simulink model "stereo_ibvs_ros2_stage1"  (R2025b)
settings: Solver=FixedStepDiscrete  StartTime=0  StopTime=inf  FixedStep=cfg.Ts  RelTol=1e-3
PostLoadFcn:
  | wrapperFile__=get_param(bdroot,'FileName');ros2Dir__=fileparts(wrapperFile__);simulinkDir__=fileparts(ros2Dir__);coreDir__=fullfile(simulinkDir__,'core');configDir__=fullfile(simulinkDir__,'config');addpath(coreDir__);addpath(configDir__);run(fullfile(configDir__,'stereo_ibvs_config.m'));clear wrapperFile__ ros2Dir__ simulinkDir__ coreDir__ configDir__;
InitFcn:
  | wrapperFile__=get_param(bdroot,'FileName');ros2Dir__=fileparts(wrapperFile__);simulinkDir__=fileparts(ros2Dir__);coreDir__=fullfile(simulinkDir__,'core');configDir__=fullfile(simulinkDir__,'config');addpath(coreDir__);addpath(configDir__);run(fullfile(configDir__,'stereo_ibvs_config.m'));clear wrapperFile__ ros2Dir__ simulinkDir__ coreDir__ configDir__;
undefined symbols (not defined in the file): cfg, data, data_SL_Info
libraries: ros2lib x10, simulink x3
settings Model: Creator=hlc  LastModifiedBy=hlc
settings DataIOCC: SignalLogging=off  SaveTime=off

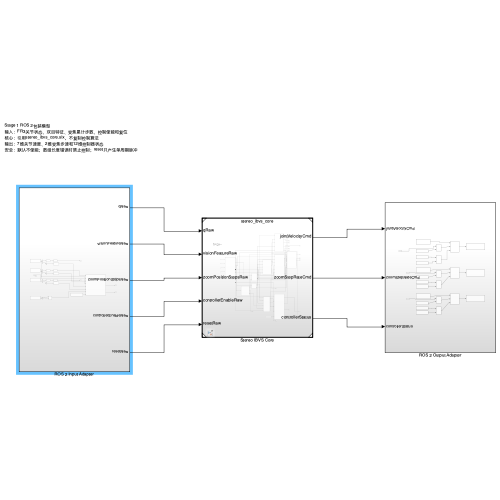
[thumbnail: Simulink's stored preview of the top-level diagram]
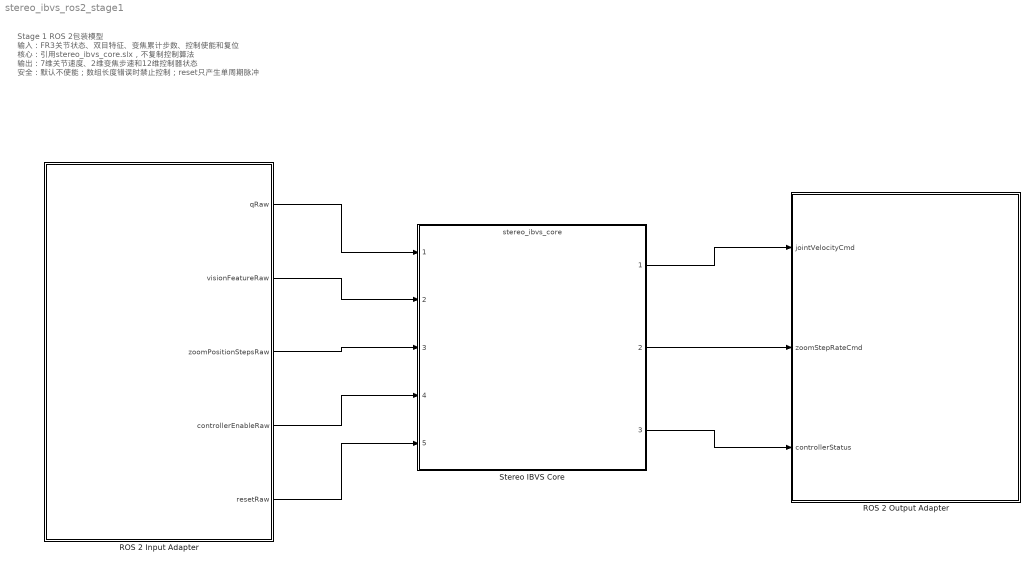
== system stereo_ibvs_ros2_stage1 ==
  note: Stage 1 ROS 2包装模型
      | 输入：FR3关节状态、双目特征、变焦累计步数、控制使能和复位
      | 核心：引用stereo_ibvs_core.slx，不复制控制算法
      | 输出：7维关节速度、2维变焦步速和12维控制器状态
      | 安全：默认不使能；数组长度错误时禁止控制；reset只产生单周期脉冲
  ROS 2 Input Adapter : Subsystem
  ROS 2 Output Adapter : Subsystem
  Stereo IBVS Core : ModelReference  ModelNameDialog=stereo_ibvs_core  SimulationMode=Normal  ModelReferenceVersion=1.49
  wires:
  ROS 2 Input Adapter/1(qRaw) -> Stereo IBVS Core/1
  ROS 2 Input Adapter/2(visionFeatureRaw) -> Stereo IBVS Core/2
  ROS 2 Input Adapter/3(zoomPositionStepsRaw) -> Stereo IBVS Core/3
  ROS 2 Input Adapter/4(controllerEnableRaw) -> Stereo IBVS Core/4
  ROS 2 Input Adapter/5(resetRaw) -> Stereo IBVS Core/5
  Stereo IBVS Core/1 -> ROS 2 Output Adapter/1(jointVelocityCmd)
  Stereo IBVS Core/2 -> ROS 2 Output Adapter/2(zoomStepRateCmd)
  Stereo IBVS Core/3 -> ROS 2 Output Adapter/3(controllerStatus)

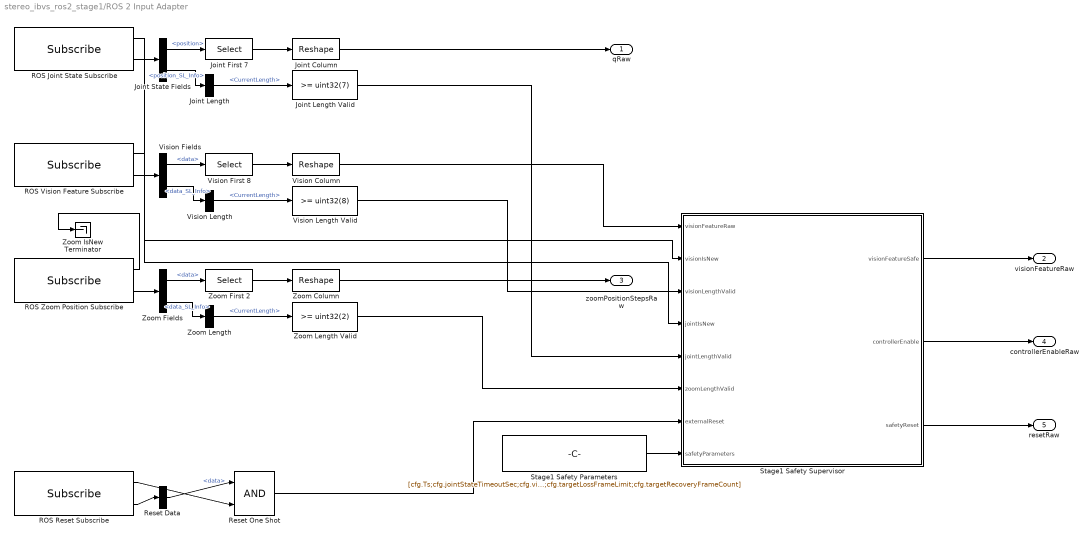
== system stereo_ibvs_ros2_stage1/ROS 2 Input Adapter ==
  Joint Column : Reshape  OutputDimensionality=Customize  OutputDimensions=[7 1]
  Joint First 7 : Selector  InputPortWidth=128  IndexOptions=Index vector (dialog)  Indices=1:7  OutputSizes=1
  Joint Length : BusSelector  OutputSignals=CurrentLength
  Joint Length Valid : simulink/Logic and Bit Operations/Compare To Constant  relop=>=  const=uint32(7)  OutDataTypeStr=boolean
  Joint State Fields : BusSelector  OutputSignals=position,position_SL_Info
  ROS Joint State Subscribe : ros2lib/Subscribe  topicSource=Specify your own  topic=/franka/joint_states  messageType=sensor_msgs/JointState  sampleTime=cfg.Ts  QOSHistory=Keep last  QOSDepth=10  QOSReliability=Reliable  QOSDurability=Volatile  QOSDeadline=Inf  QOSLifespan=Inf  QOSLiveliness=Automatic  QOSLeaseDuration=Inf  QOSAvoidROSNamespaceConventions=off
  ROS Reset Subscribe : ros2lib/Subscribe  topicSource=Specify your own  topic=/simulink/reset  messageType=std_msgs/Bool  sampleTime=cfg.Ts  QOSHistory=Keep last  QOSDepth=10  QOSReliability=Reliable  QOSDurability=Volatile  QOSDeadline=Inf  QOSLifespan=Inf  QOSLiveliness=Automatic  QOSLeaseDuration=Inf  QOSAvoidROSNamespaceConventions=off
  ROS Vision Feature Subscribe : ros2lib/Subscribe  topicSource=Specify your own  topic=/vision_double/target_features  messageType=std_msgs/Float64MultiArray  sampleTime=cfg.Ts  QOSHistory=Keep last  QOSDepth=10  QOSReliability=Reliable  QOSDurability=Volatile  QOSDeadline=Inf  QOSLifespan=Inf  QOSLiveliness=Automatic  QOSLeaseDuration=Inf  QOSAvoidROSNamespaceConventions=off
  ROS Zoom Position Subscribe : ros2lib/Subscribe  topicSource=Specify your own  topic=/vision_double/zoom_position_steps  messageType=std_msgs/Float64MultiArray  sampleTime=cfg.Ts  QOSHistory=Keep last  QOSDepth=10  QOSReliability=Reliable  QOSDurability=Volatile  QOSDeadline=Inf  QOSLifespan=Inf  QOSLiveliness=Automatic  QOSLeaseDuration=Inf  QOSAvoidROSNamespaceConventions=off
  Reset Data : BusSelector  OutputSignals=data
  Reset One Shot : Logic  AllPortsSameDT=off  OutDataTypeStr=boolean
  Stage1 Safety Parameters : Constant  Value=[cfg.Ts;cfg.jointStateTimeoutSec;cfg.visionTimeoutSec;cfg.targetLossFrameLimit;cfg.targetRecoveryFrameCount]  VectorParams1D=off  OutDataTypeStr=double  SampleTime=cfg.Ts
  Stage1 Safety Supervisor : MATLAB Function  TreatAsAtomicUnit=on
      settings: AttributesFormatString=左相机validL：连续3帧丢失后停机\nJoint/Vision：0.10 s freshness\n恢复：连续3帧有效
  Vision Column : Reshape  OutputDimensionality=Customize  OutputDimensions=[8 1]
  Vision Fields : BusSelector  OutputSignals=data,data_SL_Info
  Vision First 8 : Selector  InputPortWidth=128  IndexOptions=Index vector (dialog)  Indices=1:8  OutputSizes=1
  Vision Length : BusSelector  OutputSignals=CurrentLength
  Vision Length Valid : simulink/Logic and Bit Operations/Compare To Constant  relop=>=  const=uint32(8)  OutDataTypeStr=boolean
  Zoom Column : Reshape  OutputDimensionality=Customize  OutputDimensions=[2 1]
  Zoom Fields : BusSelector  OutputSignals=data,data_SL_Info
  Zoom First 2 : Selector  InputPortWidth=128  IndexOptions=Index vector (dialog)  Indices=1:2  OutputSizes=1
  Zoom IsNew Terminator : Terminator
  Zoom Length : BusSelector  OutputSignals=CurrentLength
  Zoom Length Valid : simulink/Logic and Bit Operations/Compare To Constant  relop=>=  const=uint32(2)  OutDataTypeStr=boolean
  qRaw : Outport  PortDimensions=[7 1]
  visionFeatureRaw : Outport  Port=2  PortDimensions=[8 1]
  zoomPositionStepsRaw : Outport  Port=3  PortDimensions=[2 1]
  controllerEnableRaw : Outport  Port=4  PortDimensions=1
  resetRaw : Outport  Port=5  PortDimensions=1
  wires:
  ROS Joint State Subscribe/2 -> Joint State Fields/1
  ROS Joint State Subscribe/1 -> Stage1 Safety Supervisor/4(jointIsNew)
  Joint State Fields/1 -> Joint First 7/1  "<position>"
  Joint First 7/1 -> Joint Column/1
  Joint Column/1 -> qRaw/1
  Joint State Fields/2 -> Joint Length/1  "<position_SL_Info>"
  Joint Length/1 -> Joint Length Valid/1  "<CurrentLength>"
  ROS Vision Feature Subscribe/2 -> Vision Fields/1
  ROS Vision Feature Subscribe/1 -> Stage1 Safety Supervisor/2(visionIsNew)
  Vision Fields/1 -> Vision First 8/1  "<data>"
  Vision First 8/1 -> Vision Column/1
  Vision Fields/2 -> Vision Length/1  "<data_SL_Info>"
  Vision Length/1 -> Vision Length Valid/1  "<CurrentLength>"
  ROS Zoom Position Subscribe/2 -> Zoom Fields/1
  ROS Zoom Position Subscribe/1 -> Zoom IsNew Terminator/1
  Zoom Fields/1 -> Zoom First 2/1  "<data>"
  Zoom First 2/1 -> Zoom Column/1
  Zoom Column/1 -> zoomPositionStepsRaw/1
  Zoom Fields/2 -> Zoom Length/1  "<data_SL_Info>"
  Zoom Length/1 -> Zoom Length Valid/1  "<CurrentLength>"
  Joint Length Valid/1 -> Stage1 Safety Supervisor/5(jointLengthValid)
  Vision Length Valid/1 -> Stage1 Safety Supervisor/3(visionLengthValid)
  Zoom Length Valid/1 -> Stage1 Safety Supervisor/6(zoomLengthValid)
  ROS Reset Subscribe/2 -> Reset Data/1
  Reset Data/1 -> Reset One Shot/1  "<data>"
  ROS Reset Subscribe/1 -> Reset One Shot/2
  Reset One Shot/1 -> Stage1 Safety Supervisor/7(externalReset)
  Vision Column/1 -> Stage1 Safety Supervisor/1(visionFeatureRaw)
  Stage1 Safety Parameters/1 -> Stage1 Safety Supervisor/8(safetyParameters)
  Stage1 Safety Supervisor/1(visionFeatureSafe) -> visionFeatureRaw/1
  Stage1 Safety Supervisor/2(controllerEnable) -> controllerEnableRaw/1
  Stage1 Safety Supervisor/3(safetyReset) -> resetRaw/1

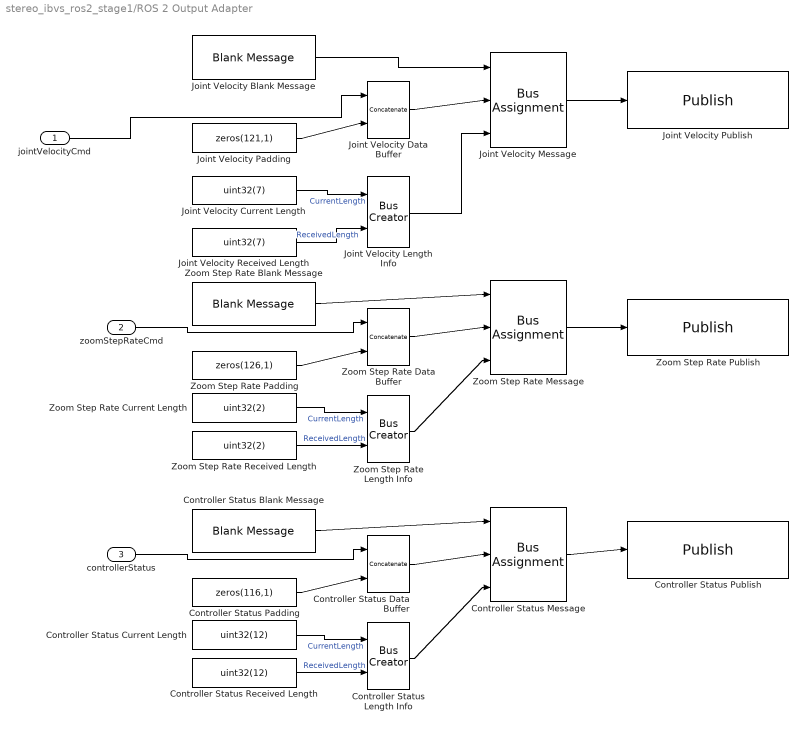
== system stereo_ibvs_ros2_stage1/ROS 2 Output Adapter ==
  jointVelocityCmd : Inport  PortDimensions=[7 1]
  zoomStepRateCmd : Inport  Port=2  PortDimensions=[2 1]
  controllerStatus : Inport  Port=3  PortDimensions=[12 1]
  Controller Status Blank Message : ros2lib/Blank Message  messageClass=Message  entityType=std_msgs/Float64MultiArray  messageType=std_msgs/Float64MultiArray  SampleTime=cfg.Ts
      link override Constant: OutDataTypeStr=Bus: SL_Bus_std_msgs_Float64MultiArray
  Controller Status Current Length : Constant  Value=uint32(12)
  Controller Status Data Buffer : Concatenate
  Controller Status Length Info : BusCreator  Inputs=2  OutDataTypeStr=Bus: SL_Bus_ROSVariableLengthArrayInfo
  Controller Status Message : BusAssignment  AssignedSignals=data,data_SL_Info
  Controller Status Padding : Constant  Value=zeros(116,1)
  Controller Status Publish : ros2lib/Publish  topicSource=Specify your own  topic=/simulink/controller_status  messageType=std_msgs/Float64MultiArray  QOSHistory=Keep last  QOSDepth=10  QOSReliability=Reliable  QOSDurability=Volatile  QOSDeadline=Inf  QOSLifespan=Inf  QOSLiveliness=Automatic  QOSLeaseDuration=Inf  QOSAvoidROSNamespaceConventions=off
  Controller Status Received Length : Constant  Value=uint32(12)
  Joint Velocity Blank Message : ros2lib/Blank Message  messageClass=Message  entityType=std_msgs/Float64MultiArray  messageType=std_msgs/Float64MultiArray  SampleTime=cfg.Ts
      link override Constant: OutDataTypeStr=Bus: SL_Bus_std_msgs_Float64MultiArray
  Joint Velocity Current Length : Constant  Value=uint32(7)
  Joint Velocity Data Buffer : Concatenate
  Joint Velocity Length Info : BusCreator  Inputs=2  OutDataTypeStr=Bus: SL_Bus_ROSVariableLengthArrayInfo
  Joint Velocity Message : BusAssignment  AssignedSignals=data,data_SL_Info
  Joint Velocity Padding : Constant  Value=zeros(121,1)
  Joint Velocity Publish : ros2lib/Publish  topicSource=Specify your own  topic=/simulink/target_joints_velocities  messageType=std_msgs/Float64MultiArray  QOSHistory=Keep last  QOSDepth=10  QOSReliability=Reliable  QOSDurability=Volatile  QOSDeadline=Inf  QOSLifespan=Inf  QOSLiveliness=Automatic  QOSLeaseDuration=Inf  QOSAvoidROSNamespaceConventions=off
  Joint Velocity Received Length : Constant  Value=uint32(7)
  Zoom Step Rate Blank Message : ros2lib/Blank Message  messageClass=Message  entityType=std_msgs/Float64MultiArray  messageType=std_msgs/Float64MultiArray  SampleTime=cfg.Ts
      link override Constant: OutDataTypeStr=Bus: SL_Bus_std_msgs_Float64MultiArray
  Zoom Step Rate Current Length : Constant  Value=uint32(2)
  Zoom Step Rate Data Buffer : Concatenate
  Zoom Step Rate Length Info : BusCreator  Inputs=2  OutDataTypeStr=Bus: SL_Bus_ROSVariableLengthArrayInfo
  Zoom Step Rate Message : BusAssignment  AssignedSignals=data,data_SL_Info
  Zoom Step Rate Padding : Constant  Value=zeros(126,1)
  Zoom Step Rate Publish : ros2lib/Publish  topicSource=Specify your own  topic=/simulink/zoom_step_rate_cmd  messageType=std_msgs/Float64MultiArray  QOSHistory=Keep last  QOSDepth=10  QOSReliability=Reliable  QOSDurability=Volatile  QOSDeadline=Inf  QOSLifespan=Inf  QOSLiveliness=Automatic  QOSLeaseDuration=Inf  QOSAvoidROSNamespaceConventions=off
  Zoom Step Rate Received Length : Constant  Value=uint32(2)
  wires:
  Joint Velocity Blank Message/1 -> Joint Velocity Message/1
  jointVelocityCmd/1 -> Joint Velocity Data Buffer/1
  Joint Velocity Padding/1 -> Joint Velocity Data Buffer/2
  Joint Velocity Data Buffer/1 -> Joint Velocity Message/2
  Joint Velocity Received Length/1 -> Joint Velocity Length Info/2  "ReceivedLength"
  Joint Velocity Length Info/1 -> Joint Velocity Message/3
  Joint Velocity Message/1 -> Joint Velocity Publish/1
  Zoom Step Rate Blank Message/1 -> Zoom Step Rate Message/1
  zoomStepRateCmd/1 -> Zoom Step Rate Data Buffer/1
  Zoom Step Rate Padding/1 -> Zoom Step Rate Data Buffer/2
  Zoom Step Rate Data Buffer/1 -> Zoom Step Rate Message/2
  Zoom Step Rate Current Length/1 -> Zoom Step Rate Length Info/1  "CurrentLength"
  Zoom Step Rate Received Length/1 -> Zoom Step Rate Length Info/2  "ReceivedLength"
  Zoom Step Rate Length Info/1 -> Zoom Step Rate Message/3
  Zoom Step Rate Message/1 -> Zoom Step Rate Publish/1
  Controller Status Blank Message/1 -> Controller Status Message/1
  controllerStatus/1 -> Controller Status Data Buffer/1
  Controller Status Padding/1 -> Controller Status Data Buffer/2
  Controller Status Data Buffer/1 -> Controller Status Message/2
  Controller Status Current Length/1 -> Controller Status Length Info/1  "CurrentLength"
  Controller Status Received Length/1 -> Controller Status Length Info/2  "ReceivedLength"
  Controller Status Length Info/1 -> Controller Status Message/3
  Controller Status Message/1 -> Controller Status Publish/1
  Joint Velocity Current Length/1 -> Joint Velocity Length Info/1  "CurrentLength"

== matlab function stereo_ibvs_ros2_stage1/ROS 2 Input Adapter/Stage1 Safety Supervisor ==
  data: visionFeatureRaw input; visionFeatureSafe output; visionIsNew input; visionLengthValid input; jointIsNew input; jointLengthValid input; zoomLengthValid input; externalReset input; safetyParameters input; controllerEnable output; safetyReset output
function [visionFeatureSafe, controllerEnable, safetyReset] = stage1SafetySupervisor(visionFeatureRaw, visionIsNew, visionLengthValid, jointIsNew, jointLengthValid, zoomLengthValid, externalReset, safetyParameters)
% 主要作用：监控JointState与视觉消息新鲜度，以左相机validL执行三帧丢失容错，并自动生成控制器使能和故障复位脉冲。
% 输入：8维视觉特征、ROS IsNew/长度状态、外部复位和5维安全参数。
% 输出：保持后的8维视觉特征、自动使能和单周期安全复位。

persistent jointAgeSec visionAgeSec jointSeen visionSeen
persistent lossCount recoveryCount enabledState
persistent heldVision heldVisionValid

sampleTime = safetyParameters(1);
jointTimeoutSec = safetyParameters(2);
visionTimeoutSec = safetyParameters(3);
lossFrameLimit = safetyParameters(4);
recoveryFrameLimit = safetyParameters(5);

if isempty(jointAgeSec)
    jointAgeSec = jointTimeoutSec + sampleTime;
    visionAgeSec = visionTimeoutSec + sampleTime;
    jointSeen = false;
    visionSeen = false;
    lossCount = 0.0;
    recoveryCount = 0.0;
    enabledState = false;
    heldVision = zeros(8,1);
    heldVisionValid = false;
end

safetyReset = 0.0;

% 人工复位同时清除安全监督器保存的上一帧和恢复计数。
if externalReset
    jointAgeSec = jointTimeoutSec + sampleTime;
    visionAgeSec = visionTimeoutSec + sampleTime;
    jointSeen = false;
    visionSeen = false;
    lossCount = 0.0;
    recoveryCount = 0.0;
    enabledState = false;
    heldVision = zeros(8,1);
    heldVisionValid = false;
    visionFeatureSafe = heldVision;
    controllerEnable = 0.0;
    safetyReset = 1.0;
    return;
end

% JointState新鲜度计时。
if jointIsNew
    jointAgeSec = 0.0;
    jointSeen = true;
else
    jointAgeSec = min(jointAgeSec + sampleTime, jointTimeoutSec + sampleTime);
end

% 视觉消息新鲜度、左相机目标丢失和合法视觉保持。
if visionIsNew
    visionAgeSec = 0.0;
    visionSeen = true;

    featureFinite = true;
    for featureIndex = 1:8
        featureFinite = featureFinite && isfinite(visionFeatureRaw(featureIndex));
    end

    leftTargetValid = visionLengthValid && featureFinite && visionFeatureRaw(1) > 0.5;

    if leftTargetValid
        heldVision = visionFeatureRaw;
        heldVisionValid = true;
        lossCount = 0.0;

        if ~enabledState
            recoveryCount = min(recoveryCount + 1.0, recoveryFrameLimit);
        end
    else
        recoveryCount = 0.0;
        lossCount = min(lossCount + 1.0, lossFrameLimit);
    end
else
    visionAgeSec = min(visionAgeSec + sampleTime, visionTimeoutSec + sampleTime);
end

jointFresh = jointSeen && jointLengthValid && jointAgeSec <= jointTimeoutSec;
visionFresh = visionSeen && visionAgeSec <= visionTimeoutSec;
zoomInputValid = zoomLengthValid;
allInputsHealthy = jointFresh && visionFresh && zoomInputValid && heldVisionValid;

previousEnabled = enabledState;

if enabledState
    if ~allInputsHealthy || lossCount >= lossFrameLimit
        enabledState = false;
        recoveryCount = 0.0;
    end
else
    if ~allInputsHealthy
        recoveryCount = 0.0;
    elseif recoveryCount >= recoveryFrameLimit
        enabledState = true;
        lossCount = 0.0;
    end
end

% 从允许运动切换到停止时，只产生一个采样周期的复位脉冲。
safetyReset = double(previousEnabled && ~enabledState);

if heldVisionValid
    visionFeatureSafe = heldVision;
else
    visionFeatureSafe = zeros(8,1);
end

controllerEnable = double(enabledState);
end
